simulink model "ex_1_RLC"  (R2018a)
settings: Solver=VariableStepAuto  StartTime=0.0  StopTime=25  MaxStep=1e-3  RelTol=1e-3
libraries: simulink x1
settings Model: Creator=k2202936  LastModifiedBy=k2202936

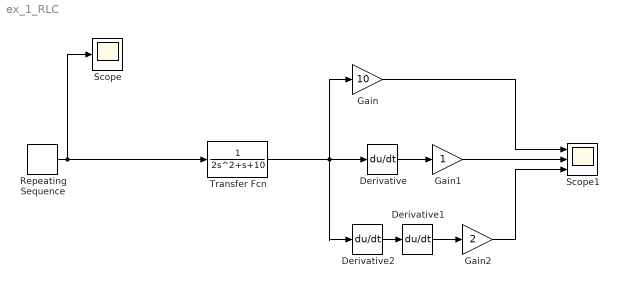
== system ex_1_RLC ==
  Derivative : Derivative
  Derivative1 : Derivative
  Derivative2 : Derivative
  Gain : Gain  Gain=10
  Gain1 : Gain
  Gain2 : Gain  Gain=2
  Repeating Sequence : simulink/Sources/Repeating Sequence  rep_seq_t=[0 5]  rep_seq_y=[0 10]
  Scope : Scope
  Scope1 : Scope  NumInputPorts=3
  Transfer Fcn : TransferFcn  Denominator=[2 1 10]
  wires:
  Repeating Sequence/1 -> Transfer Fcn/1, Scope/1
  Gain/1 -> Scope1/1
  Derivative/1 -> Gain1/1
  Transfer Fcn/1 -> Derivative2/1, Gain/1, Derivative/1
  Derivative1/1 -> Gain2/1
  Derivative2/1 -> Derivative1/1
  Gain1/1 -> Scope1/2
  Gain2/1 -> Scope1/3
